simulink model "ARI_26_3_motor_antena_nonlin_saturace_ZV"  (Simulink 7.8)
settings: Solver=ode45  StartTime=0.0  StopTime=10.0  RelTol=1e-3
undefined symbols (not defined in the file or in its folder): A, B, C, D
libraries: simulink x1
settings Model: Creator=Michael Sebek  ModifiedByFormat=Michael Sebek  LastModifiedBy=Michael Sebek
settings OptimizationCC: InitFltsAndDblsToZero=on
settings DebuggingCC: SaveWithParameterizedLinksMsg=none  SignalResolutionControl=TryResolveAllWithWarning  MultiTaskDSMMsg=warning  MultiTaskCondExecSysMsg=none  FcnCallInpInsideContextMsg=Use local settings  StrictBusMsg=None
settings RTWCC: IncludeERTFirstTime=on
settings GRTTargetCC: TargetFcnLib=ansi_tfl_tmw.mat

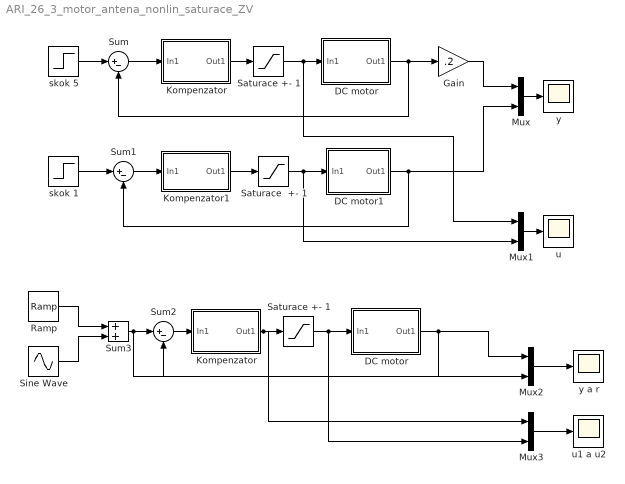
== system ARI_26_3_motor_antena_nonlin_saturace_ZV ==
  DC motor : Subsystem  mask(PMF Block){F=1/s/(s+1), InCon=[ ], SampTime=1, fvar=No change}
      mask prompts: F "PMF Object:"; InCon "Initial states:"; SampTime "Sample time (discrete time only):"; fvar "Force variable:"
      mask help:
      | Polynomial matrix fraction description of a linear system.
      |
      | This block represents a linear system defined by the polynomial matrix fraction of its transfer function.
      mask init:
      | Label = 'xxx';
      | [A,B,C,D,Label,var] = polymask2(F, fvar, length(InCon));
      | update;
      mask Help:
      | This block represents a linear system [<I>A,B,C,D</I>] defined by the polynomial matrix fraction (<I>PMF</I>) of its transfer function <I>T</I>.
      | <p>
      | <b>Left Matrix Fraction</b> item of the popup menu <b>Type</b> indicates the transfer function in the form of <I>left PMF</I>:
      | <p>
      | <I>T</I> = inv(<I>Q</I>) <I>P</I>.
      | <p>
      | <b>Right Matrix Fraction</b> item is used if the transfer function is given in the form of <I>right PMF</I>:
      | <p>
      | <I>T</I> = <I>P</I> inv(<I>Q</I>).
      | <p>
      |  The <b>variable</b> determines the type  of the system:
      | <p>
      | - <b>s, p</b> are used for continous time systems (Laplace transform).
      | <p>
      | - <b>z, q</b> are used for discrete time transfer functions in forward-shift operator (Z-transform).
      | <p>
      | - <b>d, z^-1</b> are used for discrete time transfer functions in backward-shift operator.
      | <p>
      | <b> Note:</b> For the variables <I>s,p,z,q</I>, the transfer function is defined as
      | <p>
      | <I>T</I> = <I>C</I> inv(<I>vI-A</I>) <I>B</I> + <I>D</I>,
      | <p>
      | where <I>v</I> is the variable of <I>P,Q</I>.
      | For the variables <I>d, z^-1</I>, the transfer function is defined as
      | <p>
      | <I>T</I> = <I>C v</I> inv(<I>I-Av</I>)  <I>B</I> + <I>D</I>.
      | <p>
      | <b>Note:</b> <b>Initial states</b> concern the observer-form realization of the system as defined by LMF2S and RMF2S functions. Their number must equal the sum of column degrees of the denominator matrix <I>Q</I> in case of right PMF and the sum of row degrees of <I>Q</I> for left PMF description.
      | <p>
      | See also POL, LMF2S, RMF2S.
      mask StyleString: edit,edit,edit,popup(No change|s   (continous time)|p   (continous time)|z      (discrete time)|q      (discrete time)|d      (discrete time)|z^-1 (discrete time))
      mask Display: droots([],[0 -1],1)
  "DC motor      " : Subsystem  mask(PMF Block){F=1/s/(s+1), InCon=[ ], SampTime=1, fvar=No change}
      mask prompts: F "PMF Object:"; InCon "Initial states:"; SampTime "Sample time (discrete time only):"; fvar "Force variable:"
      mask help:
      | Polynomial matrix fraction description of a linear system.
      |
      | This block represents a linear system defined by the polynomial matrix fraction of its transfer function.
      mask init:
      | Label = 'xxx';
      | [A,B,C,D,Label,var] = polymask2(F, fvar, length(InCon));
      | update;
      mask Help:
      | This block represents a linear system [<I>A,B,C,D</I>] defined by the polynomial matrix fraction (<I>PMF</I>) of its transfer function <I>T</I>.
      | <p>
      | <b>Left Matrix Fraction</b> item of the popup menu <b>Type</b> indicates the transfer function in the form of <I>left PMF</I>:
      | <p>
      | <I>T</I> = inv(<I>Q</I>) <I>P</I>.
      | <p>
      | <b>Right Matrix Fraction</b> item is used if the transfer function is given in the form of <I>right PMF</I>:
      | <p>
      | <I>T</I> = <I>P</I> inv(<I>Q</I>).
      | <p>
      |  The <b>variable</b> determines the type  of the system:
      | <p>
      | - <b>s, p</b> are used for continous time systems (Laplace transform).
      | <p>
      | - <b>z, q</b> are used for discrete time transfer functions in forward-shift operator (Z-transform).
      | <p>
      | - <b>d, z^-1</b> are used for discrete time transfer functions in backward-shift operator.
      | <p>
      | <b> Note:</b> For the variables <I>s,p,z,q</I>, the transfer function is defined as
      | <p>
      | <I>T</I> = <I>C</I> inv(<I>vI-A</I>) <I>B</I> + <I>D</I>,
      | <p>
      | where <I>v</I> is the variable of <I>P,Q</I>.
      | For the variables <I>d, z^-1</I>, the transfer function is defined as
      | <p>
      | <I>T</I> = <I>C v</I> inv(<I>I-Av</I>)  <I>B</I> + <I>D</I>.
      | <p>
      | <b>Note:</b> <b>Initial states</b> concern the observer-form realization of the system as defined by LMF2S and RMF2S functions. Their number must equal the sum of column degrees of the denominator matrix <I>Q</I> in case of right PMF and the sum of row degrees of <I>Q</I> for left PMF description.
      | <p>
      | See also POL, LMF2S, RMF2S.
      mask StyleString: edit,edit,edit,popup(No change|s   (continous time)|p   (continous time)|z      (discrete time)|q      (discrete time)|d      (discrete time)|z^-1 (discrete time))
      mask Display: droots([],[0 -1],1)
  DC motor1 : Subsystem  mask(PMF Block){F=1/s/(s+1), InCon=[ ], SampTime=1, fvar=No change}
      mask prompts: F "PMF Object:"; InCon "Initial states:"; SampTime "Sample time (discrete time only):"; fvar "Force variable:"
      mask help:
      | Polynomial matrix fraction description of a linear system.
      |
      | This block represents a linear system defined by the polynomial matrix fraction of its transfer function.
      mask init:
      | Label = 'xxx';
      | [A,B,C,D,Label,var] = polymask2(F, fvar, length(InCon));
      | update;
      mask Help:
      | This block represents a linear system [<I>A,B,C,D</I>] defined by the polynomial matrix fraction (<I>PMF</I>) of its transfer function <I>T</I>.
      | <p>
      | <b>Left Matrix Fraction</b> item of the popup menu <b>Type</b> indicates the transfer function in the form of <I>left PMF</I>:
      | <p>
      | <I>T</I> = inv(<I>Q</I>) <I>P</I>.
      | <p>
      | <b>Right Matrix Fraction</b> item is used if the transfer function is given in the form of <I>right PMF</I>:
      | <p>
      | <I>T</I> = <I>P</I> inv(<I>Q</I>).
      | <p>
      |  The <b>variable</b> determines the type  of the system:
      | <p>
      | - <b>s, p</b> are used for continous time systems (Laplace transform).
      | <p>
      | - <b>z, q</b> are used for discrete time transfer functions in forward-shift operator (Z-transform).
      | <p>
      | - <b>d, z^-1</b> are used for discrete time transfer functions in backward-shift operator.
      | <p>
      | <b> Note:</b> For the variables <I>s,p,z,q</I>, the transfer function is defined as
      | <p>
      | <I>T</I> = <I>C</I> inv(<I>vI-A</I>) <I>B</I> + <I>D</I>,
      | <p>
      | where <I>v</I> is the variable of <I>P,Q</I>.
      | For the variables <I>d, z^-1</I>, the transfer function is defined as
      | <p>
      | <I>T</I> = <I>C v</I> inv(<I>I-Av</I>)  <I>B</I> + <I>D</I>.
      | <p>
      | <b>Note:</b> <b>Initial states</b> concern the observer-form realization of the system as defined by LMF2S and RMF2S functions. Their number must equal the sum of column degrees of the denominator matrix <I>Q</I> in case of right PMF and the sum of row degrees of <I>Q</I> for left PMF description.
      | <p>
      | See also POL, LMF2S, RMF2S.
      mask StyleString: edit,edit,edit,popup(No change|s   (continous time)|p   (continous time)|z      (discrete time)|q      (discrete time)|d      (discrete time)|z^-1 (discrete time))
      mask Display: droots([],[0 -1],1)
  Gain : Gain  Gain=.2
  Kompenzator : Subsystem  mask(PMF Block){F=5*(s+2)/(s+10), InCon=[ ], SampTime=1, fvar=No change}
      mask prompts: F "PMF Object:"; InCon "Initial states:"; SampTime "Sample time (discrete time only):"; fvar "Force variable:"
      mask help:
      | Polynomial matrix fraction description of a linear system.
      |
      | This block represents a linear system defined by the polynomial matrix fraction of its transfer function.
      mask init:
      | Label = 'xxx';
      | [A,B,C,D,Label,var] = polymask2(F, fvar, length(InCon));
      | update;
      mask Help:
      | This block represents a linear system [<I>A,B,C,D</I>] defined by the polynomial matrix fraction (<I>PMF</I>) of its transfer function <I>T</I>.
      | <p>
      | <b>Left Matrix Fraction</b> item of the popup menu <b>Type</b> indicates the transfer function in the form of <I>left PMF</I>:
      | <p>
      | <I>T</I> = inv(<I>Q</I>) <I>P</I>.
      | <p>
      | <b>Right Matrix Fraction</b> item is used if the transfer function is given in the form of <I>right PMF</I>:
      | <p>
      | <I>T</I> = <I>P</I> inv(<I>Q</I>).
      | <p>
      |  The <b>variable</b> determines the type  of the system:
      | <p>
      | - <b>s, p</b> are used for continous time systems (Laplace transform).
      | <p>
      | - <b>z, q</b> are used for discrete time transfer functions in forward-shift operator (Z-transform).
      | <p>
      | - <b>d, z^-1</b> are used for discrete time transfer functions in backward-shift operator.
      | <p>
      | <b> Note:</b> For the variables <I>s,p,z,q</I>, the transfer function is defined as
      | <p>
      | <I>T</I> = <I>C</I> inv(<I>vI-A</I>) <I>B</I> + <I>D</I>,
      | <p>
      | where <I>v</I> is the variable of <I>P,Q</I>.
      | For the variables <I>d, z^-1</I>, the transfer function is defined as
      | <p>
      | <I>T</I> = <I>C v</I> inv(<I>I-Av</I>)  <I>B</I> + <I>D</I>.
      | <p>
      | <b>Note:</b> <b>Initial states</b> concern the observer-form realization of the system as defined by LMF2S and RMF2S functions. Their number must equal the sum of column degrees of the denominator matrix <I>Q</I> in case of right PMF and the sum of row degrees of <I>Q</I> for left PMF description.
      | <p>
      | See also POL, LMF2S, RMF2S.
      mask StyleString: edit,edit,edit,popup(No change|s   (continous time)|p   (continous time)|z      (discrete time)|q      (discrete time)|d      (discrete time)|z^-1 (discrete time))
      mask Display: droots([-2],[-10],5)
  "Kompenzator      " : Subsystem  mask(PMF Block){F=5*(s+2)/(s+10), InCon=[ ], SampTime=1, fvar=No change}
      mask prompts: F "PMF Object:"; InCon "Initial states:"; SampTime "Sample time (discrete time only):"; fvar "Force variable:"
      mask help:
      | Polynomial matrix fraction description of a linear system.
      |
      | This block represents a linear system defined by the polynomial matrix fraction of its transfer function.
      mask init:
      | Label = 'xxx';
      | [A,B,C,D,Label,var] = polymask2(F, fvar, length(InCon));
      | update;
      mask Help:
      | This block represents a linear system [<I>A,B,C,D</I>] defined by the polynomial matrix fraction (<I>PMF</I>) of its transfer function <I>T</I>.
      | <p>
      | <b>Left Matrix Fraction</b> item of the popup menu <b>Type</b> indicates the transfer function in the form of <I>left PMF</I>:
      | <p>
      | <I>T</I> = inv(<I>Q</I>) <I>P</I>.
      | <p>
      | <b>Right Matrix Fraction</b> item is used if the transfer function is given in the form of <I>right PMF</I>:
      | <p>
      | <I>T</I> = <I>P</I> inv(<I>Q</I>).
      | <p>
      |  The <b>variable</b> determines the type  of the system:
      | <p>
      | - <b>s, p</b> are used for continous time systems (Laplace transform).
      | <p>
      | - <b>z, q</b> are used for discrete time transfer functions in forward-shift operator (Z-transform).
      | <p>
      | - <b>d, z^-1</b> are used for discrete time transfer functions in backward-shift operator.
      | <p>
      | <b> Note:</b> For the variables <I>s,p,z,q</I>, the transfer function is defined as
      | <p>
      | <I>T</I> = <I>C</I> inv(<I>vI-A</I>) <I>B</I> + <I>D</I>,
      | <p>
      | where <I>v</I> is the variable of <I>P,Q</I>.
      | For the variables <I>d, z^-1</I>, the transfer function is defined as
      | <p>
      | <I>T</I> = <I>C v</I> inv(<I>I-Av</I>)  <I>B</I> + <I>D</I>.
      | <p>
      | <b>Note:</b> <b>Initial states</b> concern the observer-form realization of the system as defined by LMF2S and RMF2S functions. Their number must equal the sum of column degrees of the denominator matrix <I>Q</I> in case of right PMF and the sum of row degrees of <I>Q</I> for left PMF description.
      | <p>
      | See also POL, LMF2S, RMF2S.
      mask StyleString: edit,edit,edit,popup(No change|s   (continous time)|p   (continous time)|z      (discrete time)|q      (discrete time)|d      (discrete time)|z^-1 (discrete time))
      mask Display: droots([-2],[-10],5)
  Kompenzator1 : Subsystem  mask(PMF Block){F=5*(s+2)/(s+10), InCon=[ ], SampTime=1, fvar=No change}
      mask prompts: F "PMF Object:"; InCon "Initial states:"; SampTime "Sample time (discrete time only):"; fvar "Force variable:"
      mask help:
      | Polynomial matrix fraction description of a linear system.
      |
      | This block represents a linear system defined by the polynomial matrix fraction of its transfer function.
      mask init:
      | Label = 'xxx';
      | [A,B,C,D,Label,var] = polymask2(F, fvar, length(InCon));
      | update;
      mask Help:
      | This block represents a linear system [<I>A,B,C,D</I>] defined by the polynomial matrix fraction (<I>PMF</I>) of its transfer function <I>T</I>.
      | <p>
      | <b>Left Matrix Fraction</b> item of the popup menu <b>Type</b> indicates the transfer function in the form of <I>left PMF</I>:
      | <p>
      | <I>T</I> = inv(<I>Q</I>) <I>P</I>.
      | <p>
      | <b>Right Matrix Fraction</b> item is used if the transfer function is given in the form of <I>right PMF</I>:
      | <p>
      | <I>T</I> = <I>P</I> inv(<I>Q</I>).
      | <p>
      |  The <b>variable</b> determines the type  of the system:
      | <p>
      | - <b>s, p</b> are used for continous time systems (Laplace transform).
      | <p>
      | - <b>z, q</b> are used for discrete time transfer functions in forward-shift operator (Z-transform).
      | <p>
      | - <b>d, z^-1</b> are used for discrete time transfer functions in backward-shift operator.
      | <p>
      | <b> Note:</b> For the variables <I>s,p,z,q</I>, the transfer function is defined as
      | <p>
      | <I>T</I> = <I>C</I> inv(<I>vI-A</I>) <I>B</I> + <I>D</I>,
      | <p>
      | where <I>v</I> is the variable of <I>P,Q</I>.
      | For the variables <I>d, z^-1</I>, the transfer function is defined as
      | <p>
      | <I>T</I> = <I>C v</I> inv(<I>I-Av</I>)  <I>B</I> + <I>D</I>.
      | <p>
      | <b>Note:</b> <b>Initial states</b> concern the observer-form realization of the system as defined by LMF2S and RMF2S functions. Their number must equal the sum of column degrees of the denominator matrix <I>Q</I> in case of right PMF and the sum of row degrees of <I>Q</I> for left PMF description.
      | <p>
      | See also POL, LMF2S, RMF2S.
      mask StyleString: edit,edit,edit,popup(No change|s   (continous time)|p   (continous time)|z      (discrete time)|q      (discrete time)|d      (discrete time)|z^-1 (discrete time))
      mask Display: droots([-2],[-10],5)
  Mux{,1..3} (4 alike) : Mux  Inputs=2
  Ramp : simulink/Sources/Ramp  slope=.9  start=0  X0=0
  Saturace  +- 1 : Saturate  UpperLimit=1  LowerLimit=-1
  Saturace +- 1 : Saturate  UpperLimit=1  LowerLimit=-1
  "Saturace +- 1     " : Saturate  UpperLimit=1  LowerLimit=-1
  Sine Wave : Sin  Amplitude=.5  Frequency=10  SampleTime=0
  Sum : Sum  Inputs=|+-
  Sum1 : Sum  Inputs=|+-
  Sum2 : Sum  Inputs=|+-
  Sum3 : Sum
  skok 1 : Step  Time=0  SampleTime=0
  skok 5 : Step  Time=0  After=5  SampleTime=0
  u : Scope
  "u1 a u2 " : Scope
      settings: SaveName=ScopeData2
  y : Scope
  y a r : Scope
      settings: SaveName=ScopeData3
  wires:
  DC motor/1(Out1) -> Sum/2, Gain/1
  Mux/1 -> y/1
  Saturace +- 1/1 -> DC motor/1(In1), Mux1/1
  Kompenzator/1(Out1) -> Saturace +- 1/1
  Sum/1 -> Kompenzator/1(In1)
  Gain/1 -> Mux/1
  DC motor1/1(Out1) -> Sum1/2, Mux/2
  Saturace  +- 1/1 -> DC motor1/1(In1), Mux1/2
  skok 1/1 -> Sum1/1
  Sum1/1 -> Kompenzator1/1(In1)
  Kompenzator1/1(Out1) -> Saturace  +- 1/1
  Mux1/1 -> u/1
  "DC motor      "/1(Out1) -> Sum2/2, Mux2/1
  Mux2/1 -> y a r/1
  "Saturace +- 1     "/1 -> "DC motor      "/1(In1), Mux3/2
  "Kompenzator      "/1(Out1) -> "Saturace +- 1     "/1, Mux3/1
  Sum3/1 -> Sum2/1, Mux2/2
  Sum2/1 -> "Kompenzator      "/1(In1)
  Mux3/1 -> "u1 a u2 "/1
  Sine Wave/1 -> Sum3/2
  Ramp/1 -> Sum3/1
  skok 5/1 -> Sum/1

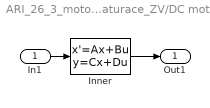
== system ARI_26_3_motor_antena_nonlin_saturace_ZV/DC motor ==
  In1 : Inport
  Inner : StateSpace  A=A  B=B  C=C  D=D  X0=InCon
  Out1 : Outport
  wires:
  Inner/1 -> Out1/1
  In1/1 -> Inner/1

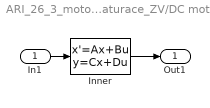
== system ARI_26_3_motor_antena_nonlin_saturace_ZV/DC motor       ==
  In1 : Inport
  Inner : StateSpace  A=A  B=B  C=C  D=D  X0=InCon
  Out1 : Outport
  wires:
  In1/1 -> Inner/1
  Inner/1 -> Out1/1

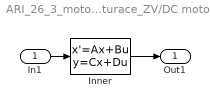
== system ARI_26_3_motor_antena_nonlin_saturace_ZV/DC motor1 ==
  In1 : Inport
  Inner : StateSpace  A=A  B=B  C=C  D=D  X0=InCon
  Out1 : Outport
  wires:
  In1/1 -> Inner/1
  Inner/1 -> Out1/1

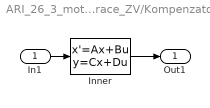
== system ARI_26_3_motor_antena_nonlin_saturace_ZV/Kompenzator ==
  In1 : Inport
  Inner : StateSpace  A=A  B=B  C=C  D=D  X0=InCon
  Out1 : Outport
  wires:
  In1/1 -> Inner/1
  Inner/1 -> Out1/1

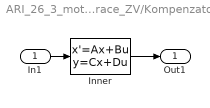
== system ARI_26_3_motor_antena_nonlin_saturace_ZV/Kompenzator       ==
  In1 : Inport
  Inner : StateSpace  A=A  B=B  C=C  D=D  X0=InCon
  Out1 : Outport
  wires:
  Inner/1 -> Out1/1
  In1/1 -> Inner/1

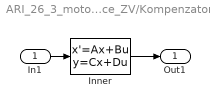
== system ARI_26_3_motor_antena_nonlin_saturace_ZV/Kompenzator1 ==
  In1 : Inport
  Inner : StateSpace  A=A  B=B  C=C  D=D  X0=InCon
  Out1 : Outport
  wires:
  Inner/1 -> Out1/1
  In1/1 -> Inner/1
